simulink model "pneumatic_tank"  (R2021a)
settings: Solver=VariableStepAuto  StartTime=0.0  StopTime=10  RelTol=1e-3
model workspace (MATLAB code in the model file):
  | V = 0.4; %liter
  | alpha = 1.5/3;
  | p_s = 6; % bar
settings Model: Creator=kjartan  LastModifiedBy=kjartan
settings SolverCC: AlgebraicLoopSolver=TrustRegion
settings DataIOCC: ReturnWorkspaceOutputs=off
settings DebuggingCC: SFMachineParentedDataDiag=warning  ArithmeticOperatorsInVariantConditions=warning
settings SFSimCC: CustomCodeUndefinedFunction=UseInterfaceOnly

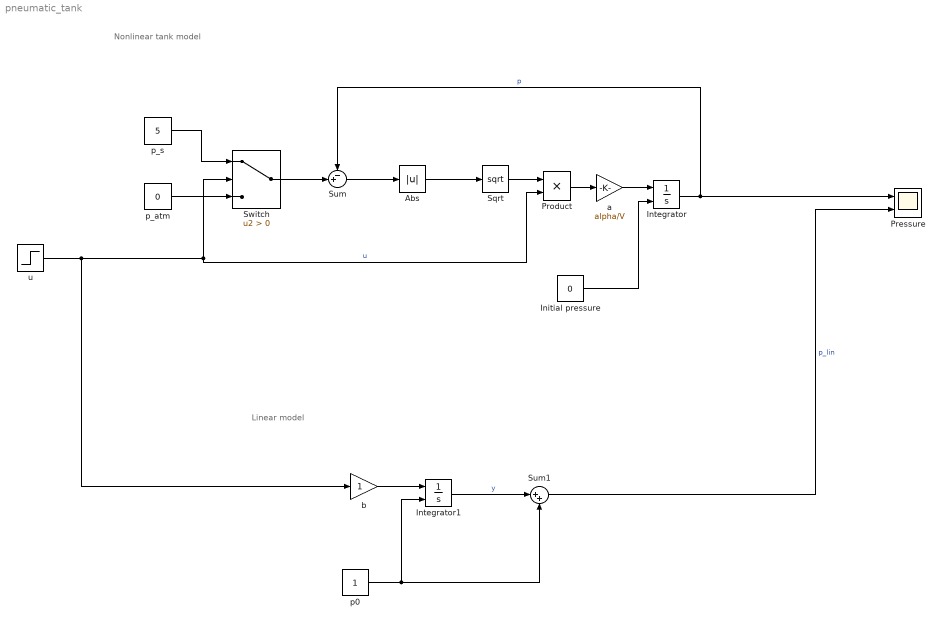
== system pneumatic_tank ==
  note: Linear model
  note: Nonlinear tank model
  Abs : Abs
  Initial pressure : Constant  Value=0  OutDataTypeStr=Inherit: Inherit via back propagation
  Integrator : Integrator  InitialConditionSource=external  InitialCondition=1  LimitOutput=on  LowerSaturationLimit=0
  Integrator1 : Integrator  InitialConditionSource=external
  Pressure : Scope  NumInputPorts=2
  Product : Product
  Sqrt : Sqrt  SaturateOnIntegerOverflow=on
  Sum : Sum  Inputs=-+|
  Sum1 : Sum  Inputs=|++
  Switch : Switch  Criteria=u2 > Threshold
  a : Gain  Gain=alpha/V
  b : Gain
  p0 : Constant
  p_atm : Constant  Value=0
  p_s : Constant  Value=5
  u : Step  Time=5  Before=3  After=-3  SampleTime=0
  wires:
  Integrator/1 -> Sum/1, Pressure/1  "p"
  Sum/1 -> Abs/1
  u/1 -> b/1, Product/2, Switch/2  "u"
  a/1 -> Integrator/1
  Product/1 -> a/1
  p_s/1 -> Switch/1
  p_atm/1 -> Switch/3
  Switch/1 -> Sum/2
  Sqrt/1 -> Product/1
  Initial pressure/1 -> Integrator/2
  Abs/1 -> Sqrt/1
  b/1 -> Integrator1/1
  p0/1 -> Sum1/2, Integrator1/2
  Integrator1/1 -> Sum1/1  "y"
  Sum1/1 -> Pressure/2  "p_lin"
